simulink model "Modello_attuatore"  (R2023a)
settings: Solver=ode14x  StartTime=0.0  StopTime=3  FixedStep=dt_sim  RelTol=1e-3
values from neighbouring files (symbols this model uses):
  A1_la = 5.710000e-003    (= 0.00571)    [C1_Actuator_1_Data.m]
  A2_la = 5.710000e-003    (= 0.00571)    [C1_Actuator_1_Data.m]
  a_jetpipe_area = 0    [B2_Main_file_Double_Active_Standby_System.m]
  A_svfb = 79.12.*1E-9.*sqrt(pi)    [B2_Main_file_Double_Active_Standby_System.m]
  a_svfb0_1 = 1E-3    (= 0.001)    [B2_Main_file_Double_Active_Standby_System.m]
  a_svfb0_2 = 0    [B2_Main_file_Double_Active_Standby_System.m]
  Afl_sv = dfl_sv^2*pi/4    (= 2.01519637574e-09)    [C1_Actuator_1_Data.m]
  Ag_sv = 18e-6    (= 1.8e-05)    [C1_Actuator_1_Data.m]
  air_gap0_1 = 0    [B2_Main_file_Double_Active_Standby_System.m]
  air_gap_fault_time = 10000    [B2_Main_file_Double_Active_Standby_System.m]
  Asp_sv = 1.35e-5    (= 1.35e-05)    [C1_Actuator_1_Data.m]
  B0_sv = 0.460    (= 0.46)    [C1_Actuator_1_Data.m]
  b_airgap = 0.3    [B2_Main_file_Double_Active_Standby_System.m]
  b_fbspring = 2E-3    (= 0.002)    [B2_Main_file_Double_Active_Standby_System.m]
  b_max = 0*0.0001    (= 0)    [C1_Actuator_1_Data.m]
  beta = 800000000    [D4_Fluid.m]    (also in Rapporto_di_trasmissione.m = acos((L-t.*cos(alpha))./s))
  beta_LVDT = 0    [aggiunte.m]
  bf_sv = 0.45    [C1_Actuator_1_Data.m]
  bsp_sv = 0.25    [C1_Actuator_1_Data.m]
  C_svfb = 1    [B2_Main_file_Double_Active_Standby_System.m]
  Cdmax_sv = 0.7392    [C1_Actuator_1_Data.m]
  Cdmin_sv = 0.6428    [C1_Actuator_1_Data.m]
  CLa = 900000    [aggiunte.m]
  Csa_la = 0.02*sqrt(Ksa_la*Meq_la)    [C1_Actuator_1_Data.m]
  Del_on = 1    [B2_Main_file_Double_Active_Standby_System.m]
  demag0_1 = 0    [B2_Main_file_Double_Active_Standby_System.m]
  dfl_sv = 5.0654e-5    (= 5.0654e-05)    [C1_Actuator_1_Data.m]
  dt_sim = 1e-5    (= 1e-05)    [B2_Main_file_Double_Active_Standby_System.m]
  enable_jetpipe_distorsion = 0    [B2_Main_file_Double_Active_Standby_System.m]
  F_att_sv = 4    [C1_Actuator_1_Data.m]
  FH = FH+0.175*pi*Dd_se(ii)*(-0.884+0.0206*Hs_se(ii)-0.0001*(Hs_se(ii))^2)*Tw_se(ii)    [D2_Data_seal.m]
  first_cycle = 0    [B2_Main_file_Double_Active_Standby_System.m]
  flight_hours = 8    [B2_Main_file_Double_Active_Standby_System.m]
  g_sv = G_sv/l0_sv    (= 0)    [C1_Actuator_1_Data.m]
  Gamma_la = 1.667e4    (= 16670)    [C1_Actuator_1_Data.m]
  gap_ms = 0    [C1_Actuator_1_Data.m]
  Gq_sv = 0.069    [C1_Actuator_1_Data.m]
  Gust_stiffness_jetpipe = 1e8    (= 100000000)    [B2_Main_file_Double_Active_Standby_System.m]
  Gust_threshold = 10000    [B2_Main_file_Double_Active_Standby_System.m]
  h_fbspring = 1E-3    (= 0.001)    [B2_Main_file_Double_Active_Standby_System.m]
  h_sv = H_sv/l0_sv    (= 0)    [C1_Actuator_1_Data.m]
  hr_sv = 6e-6    (= 6e-06)    [C1_Actuator_1_Data.m]
  hyd_fluid_repl = 20    [B2_Main_file_Double_Active_Standby_System.m]
  imax_sv = 8e-3    (= 0.008)    [C1_Actuator_1_Data.m]
  Ja_sv = 1.0575e-5    (= 1.0575e-05)    [C1_Actuator_1_Data.m]
  jetpipe_initialpos = 0    [B2_Main_file_Double_Active_Standby_System.m]
  jetpipe_passage_area = 1    [B2_Main_file_Double_Active_Standby_System.m]
  k_airgap = 0.5/100*0.01    (= 5e-05)    [B2_Main_file_Double_Active_Standby_System.m]
  k_c0_jetpipe_area = 0*1e-1    (= 0)    [B2_Main_file_Double_Active_Standby_System.m]
  k_sv = mup_sv*Vp_sv/(2*B0_sv*l0_sv)-1    (= 16.0383594613)    [C1_Actuator_1_Data.m]
  Kf_sv = 301.6    [C1_Actuator_1_Data.m]
  KFPi = zeros(m,1)    [D2_Data_seal.m]
  Kli1 = 0    [C1_Actuator_1_Data.m]
  Kli2 = 0    [C1_Actuator_1_Data.m]
  Ksa_la = 12480000    [C1_Actuator_1_Data.m]
  Kw_sv = 14.5    [C1_Actuator_1_Data.m]
  l0_sv = 0.5e-3    (= 0.0005)    [C1_Actuator_1_Data.m]
  L_c = imax_sv    (= 0.008)    [C1_Actuator_1_Data.m]
  L_la1 = 0.059900    (= 0.0599)    [C1_Actuator_1_Data.m]
  L_la2 = 0.084800    (= 0.0848)    [C1_Actuator_1_Data.m]
  la_sv = 41e-3    (= 0.041)    [C1_Actuator_1_Data.m]
  lambda_LVDT = 0*0.005*1.5    (= 0)    [aggiunte.m]
  lf = 0.025    [C1_Actuator_1_Data.m]    (also in C2_Actuator_2_Data.m)
  LVDTsize0 = 1    [aggiunte.m]
  m_thermal = 0    [B2_Main_file_Double_Active_Standby_System.m]
  Mcyl_la = 30.425550    (= 30.42555)    [C1_Actuator_1_Data.m]
  Mrod_la = 11.313490    (= 11.31349)    [C1_Actuator_1_Data.m]
  msp_sv = 0.005    [C1_Actuator_1_Data.m]
  mua_sv = 4*pi/1e7    (= 1.25663706144e-06)    [C1_Actuator_1_Data.m]
  mup_sv = 1.1*4*pi/1e7    (= 1.38230076758e-06)    [C1_Actuator_1_Data.m]
  n1_sv = 1140    [C1_Actuator_1_Data.m]
  n2_sv = 1140    [C1_Actuator_1_Data.m]
  n_svfb = 3    [B2_Main_file_Double_Active_Standby_System.m]
  null_shift = -1+2*rand(1,1)    [B2_Main_file_Double_Active_Standby_System.m]
  null_shift_sign = -1+((-1+2*rand(1,1))>=0)*2    [B2_Main_file_Double_Active_Standby_System.m]
  OV_R1 = 0*2.344e-05    (= 0)    [C1_Actuator_1_Data.m]
  OV_R2 = 0*2.344e-05    (= 0)    [C1_Actuator_1_Data.m]
  OV_S1 = 0*2.344e-05    (= 0)    [C1_Actuator_1_Data.m]
  OV_S2 = 0*2.344e-05    (= 0)    [C1_Actuator_1_Data.m]
  P01_la = Pmean-DP_eq    [C1_Actuator_1_Data.m]
  P02_la = Pmean+DP_eq    [C1_Actuator_1_Data.m]
  perc_passage_area0_1 = 0    [B2_Main_file_Double_Active_Standby_System.m]
  Pocl_A = 0    [C1_Actuator_1_Data.m]
  Pocl_B = 0    [C1_Actuator_1_Data.m]
  Pr = 600000    [B2_Main_file_Double_Active_Standby_System.m]
  Ps = 35000000    [B2_Main_file_Double_Active_Standby_System.m]
  R_th1 = 0    [B2_Main_file_Double_Active_Standby_System.m]
  Remax_sv = 5000    [C1_Actuator_1_Data.m]
  Resistance = 1    [C1_Actuator_1_Data.m]
  rj_sv = 1e-6    (= 1e-06)    [C1_Actuator_1_Data.m]
  Rp02_svspring = 1014    [B2_Main_file_Double_Active_Standby_System.m]
  sigma_0LVDT = 0*0.01*1.5*5    (= 0)    [aggiunte.m]
  ST_AD = ceil(10000/fs_AD)/10000    [C1_Actuator_1_Data.m]
  sv_crackON1 = 0    [B2_Main_file_Double_Active_Standby_System.m]
  sv_crackON2 = 0    [B2_Main_file_Double_Active_Standby_System.m]
  T0 = 0    [aggiunte.m]
  tau_w1 = 0    [B2_Main_file_Double_Active_Standby_System.m]
  Temperature_threshold = 0    [B2_Main_file_Double_Active_Standby_System.m]
  V01_la = (Vm_la1+A1_la*(L_la1+x0_la))    (= 0.00040017393)    [C1_Actuator_1_Data.m]
  V02_la = (Vm_la2+A2_la*(L_la2-x0_la))    (= 0.00056652336)    [C1_Actuator_1_Data.m]
  Voltage_com = Resistance    (= 1)    [C1_Actuator_1_Data.m]
  Vp_sv = 5.67e3    (= 5670)    [C1_Actuator_1_Data.m]
  w_fb = 310    [C1_Actuator_1_Data.m]
  w_sv = W_sv/l0_sv    (= 0)    [C1_Actuator_1_Data.m]
  wsp_sv = 0.009334348785340    (= 0.00933434878534)    [C1_Actuator_1_Data.m]
  x0_la = 0    [C1_Actuator_1_Data.m]
  xf_sv_max = 3.05e-5    (= 3.05e-05)    [C1_Actuator_1_Data.m]
  xmax_sb = 5.5e-3    (= 0.0055)    [C1_Actuator_1_Data.m]
  xspmax_sv = 0.001250    (= 0.00125)    [C1_Actuator_1_Data.m]
  z_fb = 0.5    [C1_Actuator_1_Data.m]
undefined symbols (not defined in the file or in its folder): magnitude, Newton, R_sp_C, Raphson
libraries: simulink x13
(part 2 of 3)

== system Modello_attuatore/Actuation System/Servovalve/Spool/orifice2R-resistences ==
  In3 : Inport
  In6 : Inport  Port=2
  In4 : Inport  Port=3
  >=0 : Saturate  UpperLimit=0  LowerLimit=-inf
  >=1 : Saturate  UpperLimit=inf  LowerLimit=0
  Abs : Abs  SaturateOnIntegerOverflow=off
  Abs1 : Abs  SaturateOnIntegerOverflow=off
  Add3 : Sum  Inputs=-|+
  Add4 : Sum  Inputs=+|+
  Cd : Subsystem
  Demux : Demux  Outputs=2
  Fcn : Fcn  Expr=12*u(2)*u(1)/(2.5*wsp_sv*hr_sv^3)
  Fcn1 : Fcn  Expr=u(1)/(2*u(2)^2*u(3)^2)
  Math Function2 : Math  Operator=magnitude^2  SignedPower=on
  Math Function3 : Math  Operator=magnitude^2  SignedPower=on
  Mux : Mux  Inputs=2
  Mux1 : Mux  Inputs=3
  Product : Product  RndMeth=Zero
  Sqrt1 : Sqrt  AlgorithmType=Newton-Raphson
  gioco radiale : Constant  Value=hr_sv
  gioco radiale1 : Constant  Value=wsp_sv
  ricoprimento : Constant  Value=OV_R2
  Out1 : Outport
  Out2 : Outport  Port=2
  wires:
  Mux/1 -> Fcn/1
  Mux1/1 -> Fcn1/1
  Fcn1/1 -> Out1/1  "R_AR2"
  Demux/2 -> Mux/2  "mu [Pa s]"
  Cd/1(Out3) -> Mux1/2  "Cd"
  In4/1 -> Abs/1  "Q2R[m3/s]"
  Demux/1 -> Mux1/1  "ro [kg/m3]"
  In6/1 -> Demux/1  "ro;mu"
  ricoprimento/1 -> Add3/1
  In3/1 -> Add3/2  "xs[m]"
  Abs/1 -> Cd/1(In2)
  gioco radiale/1 -> Math Function2/1  "hr[m]"
  Add3/1 -> >=1/1, >=0/1  "x[m]"
  >=0/1 -> Abs1/1
  Add4/1 -> Sqrt1/1
  Math Function3/1 -> Add4/1
  Math Function2/1 -> Add4/2
  gioco radiale1/1 -> Product/2  "w[m]"
  Abs1/1 -> Mux/1
  >=1/1 -> Math Function3/1, Cd/2(In1)
  Sqrt1/1 -> Product/1, Cd/3(In3)  "l[m]"
  Product/1 -> Mux1/3  "A [m2]"
  Fcn/1 -> Out2/1  "R_CR2"

== system Modello_attuatore/Actuation System/Servovalve/Spool/orifice2S-resistences ==
  In3 : Inport
  In6 : Inport  Port=2
  In4 : Inport  Port=3
  >=0 : Saturate  UpperLimit=inf  LowerLimit=0
  >=1 : Saturate  UpperLimit=0  LowerLimit=-inf
  Abs : Abs  SaturateOnIntegerOverflow=off
  Abs1 : Abs  SaturateOnIntegerOverflow=off
  Add3 : Sum  Inputs=+|+
  Add4 : Sum  Inputs=+|+
  Cd : Subsystem
  Demux : Demux  Outputs=2
  Fcn : Fcn  Expr=12*u(2)*u(1)/(2.5*wsp_sv*hr_sv^3)
  Fcn1 : Fcn  Expr=u(1)/(2*u(2)^2*u(3)^2)
  Math Function2 : Math  Operator=magnitude^2  SignedPower=on
  Math Function3 : Math  Operator=magnitude^2  SignedPower=on
  Mux : Mux  Inputs=2
  Mux1 : Mux  Inputs=3
  Product : Product  RndMeth=Zero
  Sqrt1 : Sqrt  AlgorithmType=Newton-Raphson
  gioco radiale : Constant  Value=hr_sv
  gioco radiale1 : Constant  Value=wsp_sv
  ricoprimento : Constant  Value=OV_S2
  Out1 : Outport
  Out2 : Outport  Port=2
  wires:
  Mux/1 -> Fcn/1
  Mux1/1 -> Fcn1/1
  Fcn1/1 -> Out1/1  "R_AS2"
  Demux/2 -> Mux/2  "mu [Pa s]"
  Cd/1(Out3) -> Mux1/2  "Cd"
  In4/1 -> Abs/1  "Q2S[m3/s]"
  Demux/1 -> Mux1/1  "ro [kg/m3]"
  In6/1 -> Demux/1  "ro;mu"
  ricoprimento/1 -> Add3/1
  In3/1 -> Add3/2  "xs[m]"
  Abs/1 -> Cd/1(In2)
  gioco radiale/1 -> Math Function2/1  "hr[m]"
  Add3/1 -> >=1/1, >=0/1  "x[m]"
  >=0/1 -> Abs1/1
  Add4/1 -> Sqrt1/1
  Math Function3/1 -> Add4/1
  Math Function2/1 -> Add4/2
  gioco radiale1/1 -> Product/2  "w[m]"
  Abs1/1 -> Mux/1
  >=1/1 -> Math Function3/1, Cd/2(In1)
  Sqrt1/1 -> Product/1, Cd/3(In3)  "l[m]"
  Product/1 -> Mux1/3  "A [m2]"
  Fcn/1 -> Out2/1  "R_CS2"

== system Modello_attuatore/Actuation System/Servovalve/Spool/orificeS1-flow ==
  In4 : Inport
  In2 : Inport  Port=2
  In1 : Inport  Port=3
  Gain : Gain  Gain=4  SaturateOnIntegerOverflow=on  OutDataTypeStr=Inherit: Same as input  ParamDataTypeStr=Inherit: Same as input
  Gain1 : Gain  Gain=2  SaturateOnIntegerOverflow=on  OutDataTypeStr=Inherit: Same as input  ParamDataTypeStr=Inherit: Same as input
  Math Function : Math  Operator=sqrt  SignedPower=on
  Math Function1 : Math  Operator=magnitude^2  SignedPower=on
  Product : Product  Inputs=3  SaturateOnIntegerOverflow=on  OutDataTypeStr=Inherit: Same as first input
  Product1 : Product  Inputs=*/  SaturateOnIntegerOverflow=on  OutDataTypeStr=Inherit: Same as first input
  Product2 : Product  SaturateOnIntegerOverflow=on  OutDataTypeStr=Inherit: Same as first input
  Sign : Signum
  Sum : Sum  Inputs=|++  SaturateOnIntegerOverflow=on
  Sum1 : Sum  Inputs=|+-  SaturateOnIntegerOverflow=on
  Out1 : Outport
  wires:
  Sign/1 -> Product/1, Product2/1
  In4/1 -> Product/2, Sign/1  "dP[Pa]"
  In2/1 -> Gain1/1, Product/3  "R_AS1"
  Product/1 -> Gain/1
  Gain/1 -> Sum/1
  Math Function1/1 -> Sum/2
  Sum/1 -> Math Function/1
  Math Function/1 -> Sum1/1
  Sum1/1 -> Product1/1
  Gain1/1 -> Product1/2
  Product1/1 -> Product2/2
  In1/1 -> Sum1/2, Math Function1/1  "R_CS1"
  Product2/1 -> Out1/1  "Q_1S[m3/s]"

== system Modello_attuatore/Actuation System/Servovalve/Spool/orificeS2-flow ==
  In4 : Inport
  In1 : Inport  Port=2
  In2 : Inport  Port=3
  Gain : Gain  Gain=4  SaturateOnIntegerOverflow=on  OutDataTypeStr=Inherit: Same as input  ParamDataTypeStr=Inherit: Same as input
  Gain1 : Gain  Gain=2  SaturateOnIntegerOverflow=on  OutDataTypeStr=Inherit: Same as input  ParamDataTypeStr=Inherit: Same as input
  Math Function : Math  Operator=sqrt  SignedPower=on
  Math Function1 : Math  Operator=magnitude^2  SignedPower=on
  Product : Product  Inputs=3  SaturateOnIntegerOverflow=on  OutDataTypeStr=Inherit: Same as first input
  Product1 : Product  Inputs=*/  SaturateOnIntegerOverflow=on  OutDataTypeStr=Inherit: Same as first input
  Product2 : Product  SaturateOnIntegerOverflow=on  OutDataTypeStr=Inherit: Same as first input
  Sign : Signum
  Sum : Sum  Inputs=|++  SaturateOnIntegerOverflow=on
  Sum1 : Sum  Inputs=|+-  SaturateOnIntegerOverflow=on
  Out4 : Outport
  wires:
  Product2/1 -> Out4/1  "Q_2S[m3/s]"
  In2/1 -> Math Function1/1, Sum1/2  "R_CR2"
  Product1/1 -> Product2/2
  Gain1/1 -> Product1/2
  Sum1/1 -> Product1/1
  Math Function/1 -> Sum1/1
  Sum/1 -> Math Function/1
  Math Function1/1 -> Sum/2
  Gain/1 -> Sum/1
  Product/1 -> Gain/1
  In1/1 -> Product/3, Gain1/1  "R_AS2"
  In4/1 -> Product/2, Sign/1  "dP[Pa]"
  Sign/1 -> Product2/1, Product/1

== system Modello_attuatore/Actuation System/Actuator/Rod/Double Integrator/Limit ==
  In2 : Inport
  In1 : Inport  Port=2
  Constant : Constant
  Constant1 : Constant  Value=-1
  Constant2 : Constant  Value=0
  Constant3 : Constant  Value=0
  Logical Operator : Logic  AllPortsSameDT=off
  Logical Operator1 : Logic  AllPortsSameDT=off
  Logical Operator2 : Logic  Operator=NOR  AllPortsSameDT=off
  Product : Product  RndMeth=Zero
  Relational Operator : RelationalOperator  Operator=>  OutDataTypeStr=boolean  InputSameDT=off
  Relational Operator1 : RelationalOperator  Operator===  OutDataTypeStr=boolean  InputSameDT=off
  Relational Operator2 : RelationalOperator  Operator=<  OutDataTypeStr=boolean  InputSameDT=off
  Relational Operator3 : RelationalOperator  Operator===  OutDataTypeStr=boolean  InputSameDT=off
  Out2 : Outport
  wires:
  In2/1 -> Relational Operator/1, Product/1, Relational Operator2/1  "xrod_dd [m/s2]"
  In1/1 -> Relational Operator3/1, Relational Operator1/1  "limit xrod"
  Constant3/1 -> Relational Operator/2
  Constant/1 -> Relational Operator1/2
  Constant1/1 -> Relational Operator3/2
  Constant2/1 -> Relational Operator2/2
  Relational Operator/1 -> Logical Operator/1
  Relational Operator1/1 -> Logical Operator/2
  Relational Operator3/1 -> Logical Operator1/1
  Relational Operator2/1 -> Logical Operator1/2
  Logical Operator/1 -> Logical Operator2/1
  Logical Operator1/1 -> Logical Operator2/2
  Logical Operator2/1 -> Product/2
  Product/1 -> Out2/1  "xrod_dd [m2/s]"

== system Modello_attuatore/Actuation System/Actuator/Rod/Friction1/FP ==
  In3 : Inport
  Abs : Abs  SaturateOnIntegerOverflow=off
  Abs1 : Abs  SaturateOnIntegerOverflow=off
  Abs2 : Abs  SaturateOnIntegerOverflow=off
  Add1 : Sum  Inputs=+|+
  Constant1 : Constant  Value=KFPi
  Constant2 : Constant  Value=FH
  Demux : Demux  Outputs=2
  Display : Display
  Display1 : Display
  Mux6 : Mux  Inputs=2
  P1-Patm : Fcn  Expr=(u(1)*1e-6)^0.61
  P2-Patm : Fcn  Expr=(u(1)*1e-6)^0.61
  Product3 : Product  RndMeth=Zero
  Scope3 : Scope
  Scope4 : Scope
  Sum of Elements : Sum  Inputs=+
  Vector Concatenate1 : Concatenate  NumInputs=3  ConcatenateDimension=2
  abs(P1-P2) : Fcn  Expr=(abs(u(1)-u(2))*1e-6)^0.61
  Out4 : Outport
  wires:
  Constant2/1 -> Display1/1, Add1/2
  Add1/1 -> Out4/1, Scope3/1  "FP+FH"
  Sum of Elements/1 -> Add1/1, Display/1  "FP"
  Abs/1 -> abs(P1-P2)/1
  Product3/1 -> Sum of Elements/1  "KFPi"
  Constant1/1 -> Product3/2
  Vector Concatenate1/1 -> Scope4/1, Product3/1
  abs(P1-P2)/1 -> Vector Concatenate1/3
  P2-Patm/1 -> Vector Concatenate1/2
  Demux/2 -> Mux6/2, Abs2/1  "P2"
  Demux/1 -> Mux6/1, Abs1/1  "P1"
  P1-Patm/1 -> Vector Concatenate1/1
  Mux6/1 -> Abs/1
  In3/1 -> Demux/1  "P"
  Abs1/1 -> P1-Patm/1
  Abs2/1 -> P2-Patm/1

== system Modello_attuatore/Actuation System/Actuator/Sleeve/Backlash/No Backlash ==
  In1 : Inport
  In2 : Inport  Port=2
  Action Port : ActionPort  PropagateVarSize=During execution  ActionPortLabel=if(u1<=1e-10)
  Add4 : Sum  Inputs=+|+
  Cs_shaft [Nm/(rad/s)] : Gain  Gain=Csa_la
  Ks_shaft [Nm/rad] : Gain  Gain=Ksa_la
  Out3 : Outport
  wires:
  Ks_shaft [Nm/rad]/1 -> Add4/1
  Cs_shaft [Nm/(rad/s)]/1 -> Add4/2
  Add4/1 -> Out3/1
  In1/1 -> Ks_shaft [Nm/rad]/1
  In2/1 -> Cs_shaft [Nm/(rad/s)]/1

== system Modello_attuatore/Actuation System/Actuator/Sleeve/Backlash/No contact ==
  In2 : Inport
  In3 : Inport  Port=2
  Action Port : ActionPort  PropagateVarSize=During execution  ActionPortLabel=else
  Add4 : Sum  Inputs=+|+
  no torque : Gain  Gain=0
  Out3 : Outport
  wires:
  no torque/1 -> Out3/1
  In2/1 -> Add4/1
  In3/1 -> Add4/2
  Add4/1 -> no torque/1

== system Modello_attuatore/Actuation System/Actuator/Sleeve/Backlash/phi diff > max backlash ==
  In2 : Inport
  In3 : Inport  Port=2
  Action Port : ActionPort  PropagateVarSize=During execution  ActionPortLabel=elseif(u2>u3)
  Add1 : Sum  Inputs=+|-
  Add2 : Sum  Inputs=+|+
  Add4 : Sum  Inputs=+|+
  Compare To Zero : simulink/Logic and Bit Operations/Compare To Zero  relop=<=  OutDataTypeStr=uint8
  Constant : Constant  Value=0
  Constant2 : Constant  Value=b_max/2
  Cs_shaft [Nm/(rad/s)] : Gain  Gain=Csa_la
  Ks_shaft [Nm/rad] : Gain  Gain=Ksa_la
  MinMax : MinMax  Inputs=2
  Switch : Switch  Criteria=u2 > Threshold  SaturateOnIntegerOverflow=off  InputSameDT=off
  Out1 : Outport
  wires:
  Ks_shaft [Nm/rad]/1 -> Add4/1, MinMax/1, Add2/1
  Cs_shaft [Nm/(rad/s)]/1 -> Add4/2, MinMax/2
  In3/1 -> Cs_shaft [Nm/(rad/s)]/1
  In2/1 -> Add1/1
  Constant2/1 -> Add1/2
  Add1/1 -> Ks_shaft [Nm/rad]/1
  Compare To Zero/1 -> Switch/2
  Constant/1 -> Switch/1
  Add4/1 -> Compare To Zero/1
  MinMax/1 -> Add2/2
  Add2/1 -> Switch/3
  Switch/1 -> Out1/1  "Force [N]"

== system Modello_attuatore/Actuation System/Actuator/Sleeve/Backlash/phi diff< min backlash ==
  In2 : Inport
  In3 : Inport  Port=2
  Action Port : ActionPort  PropagateVarSize=During execution  ActionPortLabel=elseif( u2<u4)
  Add1 : Sum  Inputs=+|-
  Add2 : Sum  Inputs=+|+
  Add4 : Sum  Inputs=+|+
  Compare To Zero : simulink/Logic and Bit Operations/Compare To Zero  relop=>=  OutDataTypeStr=uint8
  Constant : Constant  Value=0
  Constant1 : Constant  Value=-b_max/2
  Cs_shaft [Nm/(rad/s)] : Gain  Gain=Csa_la
  Ks_shaft [Nm/rad] : Gain  Gain=Ksa_la
  MinMax : MinMax  Function=max  Inputs=2
  Switch : Switch  Criteria=u2 > Threshold  SaturateOnIntegerOverflow=off  InputSameDT=off
  Out1 : Outport
  wires:
  Ks_shaft [Nm/rad]/1 -> Add4/1, MinMax/1, Add2/1
  Cs_shaft [Nm/(rad/s)]/1 -> Add4/2, MinMax/2
  In3/1 -> Cs_shaft [Nm/(rad/s)]/1
  In2/1 -> Add1/1
  Constant1/1 -> Add1/2
  Add1/1 -> Ks_shaft [Nm/rad]/1
  Compare To Zero/1 -> Switch/2
  Constant/1 -> Switch/1
  Add4/1 -> Compare To Zero/1
  MinMax/1 -> Add2/2
  Add2/1 -> Switch/3
  Switch/1 -> Out1/1  "Force [N]"

== system Modello_attuatore/Actuation System/Servovalve/Servovalve Dynamic/Crack propagation/Bending (normal) stress computation ==
  Tb [Nm] : Inport
  Crack_size[mm] : Inport  Port=2
  Add : Sum  Inputs=-+
  Constant : Constant  Value=b_fbspring*1000
  Constant1 : Constant  Value=h_fbspring*1000
  Divide : Product  Inputs=*/*
  Divide1 : Product  Inputs=**
  Fcn : Fcn  Expr=(u(1)^3)
  Gain : Gain  Gain=0.5
  Gain1 : Gain
  Gain2 : Gain  Gain=1/12
  Gain3 : Gain  Gain=1000
  Saturation : Saturate  UpperLimit=Inf  LowerLimit=1E-5
  sigma [MPa] : Outport
  wires:
  Tb [Nm]/1 -> Gain3/1
  Add/1 -> Fcn/1, Gain/1
  Divide/1 -> Gain1/1
  Crack_size[mm]/1 -> Add/1
  Constant1/1 -> Add/2
  Gain/1 -> Divide/3
  Gain1/1 -> sigma [MPa]/1
  Fcn/1 -> Gain2/1  "Wbend"
  Gain2/1 -> Divide1/2
  Constant/1 -> Divide1/1
  Divide1/1 -> Saturation/1
  Saturation/1 -> Divide/2
  Gain3/1 -> Divide/1

== system Modello_attuatore/Actuation System/Servovalve/Servovalve Dynamic/Crack propagation/Enabled Subsystem ==
  max,min : Inport
  Enable : EnablePort  StatesWhenEnabling=reset  ShowOutputPort=on
  Abs : Abs  SaturateOnIntegerOverflow=off
  Add : Sum  Inputs=+-
  Add1 : Sum  Inputs=+-
  Demux : Demux  Outputs=2
  Saturation : Saturate  UpperLimit=inf  LowerLimit=0
  Saturation1 : Saturate  UpperLimit=0  LowerLimit=-inf
  Saturation2 : Saturate  UpperLimit=inf  LowerLimit=0
  Saturation3 : Saturate  UpperLimit=0  LowerLimit=-inf
  DeltaS_side1 : Outport
  DeltaS_side2 : Outport  Port=2
  Reset_minmax : Outport  Port=3
  wires:
  max,min/1 -> Demux/1
  Demux/2 -> Saturation/1, Saturation3/1
  Demux/1 -> Saturation1/1, Saturation2/1
  Saturation/1 -> Add/2
  Saturation2/1 -> Add/1
  Saturation3/1 -> Add1/2
  Add/1 -> DeltaS_side1/1
  Add1/1 -> Abs/1
  Enable/1 -> Reset_minmax/1
  Abs/1 -> DeltaS_side2/1
  Saturation1/1 -> Add1/1

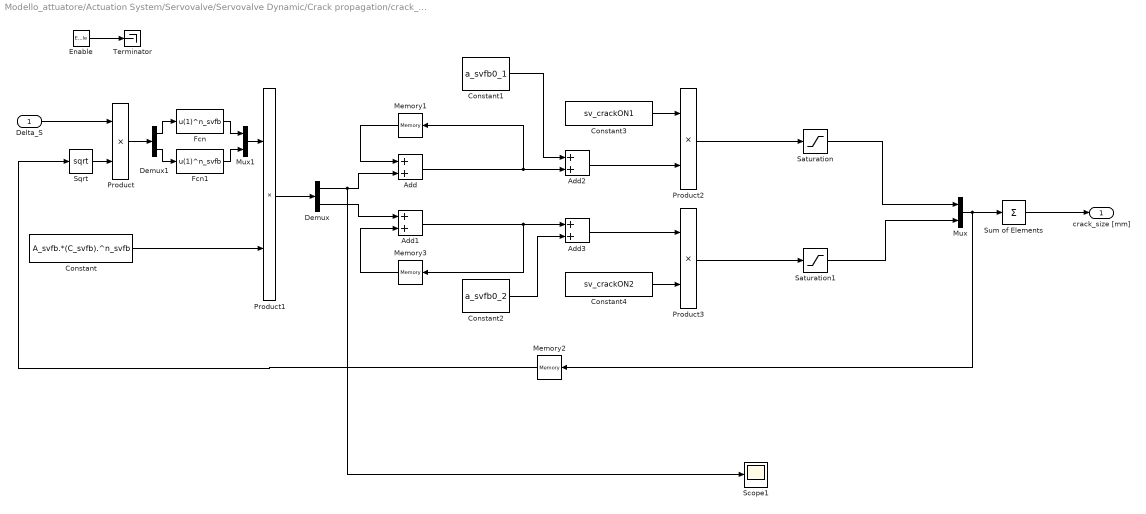
== system Modello_attuatore/Actuation System/Servovalve/Servovalve Dynamic/Crack propagation/crack_size calculation ==
  Delta_S : Inport
  Enable : EnablePort  ShowOutputPort=on
  Add{,1..3} (4 alike) : Sum
  Constant : Constant  Value=A_svfb.*(C_svfb).^n_svfb
  Constant1 : Constant  Value=a_svfb0_1
  Constant2 : Constant  Value=a_svfb0_2
  Constant3 : Constant  Value=sv_crackON1
  Constant4 : Constant  Value=sv_crackON2
  Demux : Demux  Outputs=2
  Demux1 : Demux  Outputs=2
  Fcn : Fcn  Expr=u(1)^n_svfb
  Fcn1 : Fcn  Expr=u(1)^n_svfb
  Memory1 : Memory
  Memory2 : Memory  InitialCondition=[a_svfb0_1; a_svfb0_2]
  Memory3 : Memory
  Mux : Mux  Inputs=2
  Mux1 : Mux  Inputs=2
  Product{,1..3} (4 alike) : Product
  Saturation : Saturate  UpperLimit=h_fbspring*1000  LowerLimit=0
  Saturation1 : Saturate  UpperLimit=h_fbspring*1000  LowerLimit=0
  Scope1 : Scope
  Sqrt : Sqrt
  Sum of Elements : Sum  Inputs=+
  Terminator : Terminator
  crack_size [mm] : Outport
  wires:
  Delta_S/1 -> Product/1
  Sqrt/1 -> Product/2
  Constant/1 -> Product1/2
  Product1/1 -> Demux/1
  Demux/2 -> Add1/1
  Add/1 -> Memory1/1, Add2/2
  Add1/1 -> Memory3/1, Add3/1
  Constant1/1 -> Add2/1
  Constant2/1 -> Add3/2
  Add2/1 -> Product2/2
  Constant3/1 -> Product2/1
  Constant4/1 -> Product3/2
  Add3/1 -> Product3/1
  Product2/1 -> Saturation/1
  Product3/1 -> Saturation1/1
  Product/1 -> Demux1/1
  Demux1/1 -> Fcn/1
  Demux1/2 -> Fcn1/1
  Fcn/1 -> Mux1/1
  Fcn1/1 -> Mux1/2
  Sum of Elements/1 -> crack_size [mm]/1
  Memory1/1 -> Add/1
  Memory3/1 -> Add1/2
  Mux1/1 -> Product1/1
  Mux/1 -> Memory2/1, Sum of Elements/1
  Memory2/1 -> Sqrt/1
  Saturation/1 -> Mux/1
  Saturation1/1 -> Mux/2
  Enable/1 -> Terminator/1
  Demux/1 -> Scope1/1, Add/2

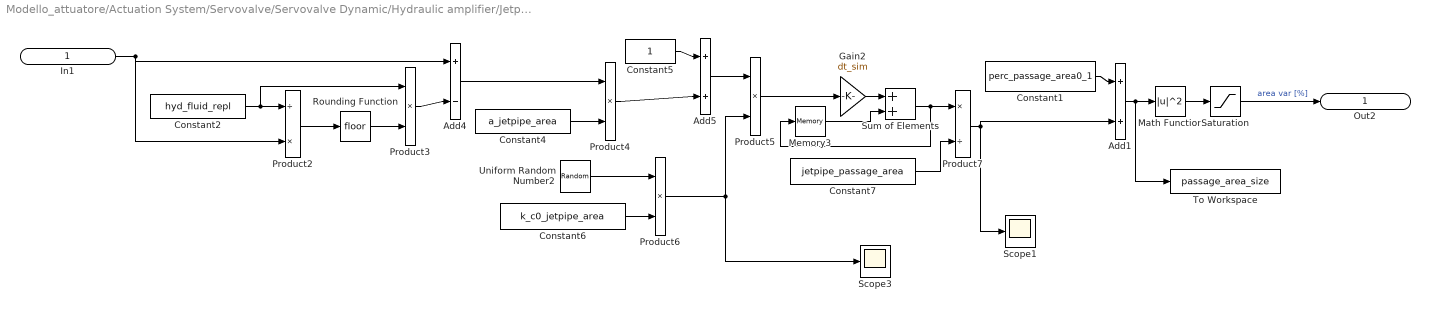
== system Modello_attuatore/Actuation System/Servovalve/Servovalve Dynamic/Hydraulic amplifier/Jetpipe area occlusion ==
  In1 : Inport
  Add1 : Sum  Inputs=+|+
  Add4 : Sum  Inputs=+|-
  Add5 : Sum  Inputs=+|+
  Constant1 : Constant  Value=perc_passage_area0_1
  Constant2 : Constant  Value=hyd_fluid_repl
  Constant4 : Constant  Value=a_jetpipe_area
  Constant5 : Constant
  Constant6 : Constant  Value=k_c0_jetpipe_area
  Constant7 : Constant  Value=jetpipe_passage_area
  Gain2 : Gain  Gain=dt_sim
  Math Function : Math  Operator=magnitude^2  SignedPower=on
  Memory3 : Memory
  Product2 : Product  Inputs=/*  SaturateOnIntegerOverflow=on  OutDataTypeStr=Inherit: Same as first input
  Product{3..6} (4 alike) : Product  SaturateOnIntegerOverflow=on  OutDataTypeStr=Inherit: Same as first input
  Product7 : Product  Inputs=*/  SaturateOnIntegerOverflow=on  OutDataTypeStr=Inherit: Same as first input
  Rounding Function : Rounding
  Saturation : Saturate  UpperLimit=0.8  LowerLimit=0
  Scope1 : Scope
  Scope3 : Scope
  Sum of Elements : Sum
  To Workspace : ToWorkspace  VariableName=passage_area_size  SaveFormat=Structure With Time  SampleTime=-1
  Uniform Random Number2 : UniformRandomNumber  Minimum=1  Maximum=5
  Out2 : Outport
  wires:
  In1/1 -> Product2/2, Add4/1
  Product2/1 -> Rounding Function/1
  Constant2/1 -> Product2/1, Product3/1
  Rounding Function/1 -> Product3/2
  Product3/1 -> Add4/2
  Add4/1 -> Product4/1
  Product4/1 -> Add5/2
  Constant5/1 -> Add5/1
  Constant4/1 -> Product4/2
  Add5/1 -> Product5/1
  Constant6/1 -> Product6/2
  Uniform Random Number2/1 -> Product6/1
  Product6/1 -> Product5/2, Scope3/1
  Gain2/1 -> Sum of Elements/1
  Product5/1 -> Gain2/1
  Sum of Elements/1 -> Memory3/1, Product7/1
  Memory3/1 -> Sum of Elements/2
  Constant7/1 -> Product7/2
  Product7/1 -> Scope1/1, Add1/2
  Saturation/1 -> Out2/1  "area var [%]"
  Add1/1 -> Math Function/1, To Workspace/1
  Constant1/1 -> Add1/1
  Math Function/1 -> Saturation/1

== system Modello_attuatore/Actuation System/Servovalve/Servovalve Dynamic/Hydraulic amplifier/Ugello A ==
  In4 : Inport
  In2 : Inport  Port=2
  In1 : Inport  Port=3
  In3 : Inport  Port=4
  In5 : Inport  Port=5
  Add1 : Sum  Inputs=+|-
  Add2 : Sum  Inputs=+|+
  Constant : Fcn  Expr=((u(2)-(u(4)*u(2)))-(u(3)+Pocl_A))/2+(u(3)+Pocl_A)
  Gain1 : Gain  Gain=Asp_sv/Gq_sv
  Mux2 : Mux
  Saturation2 : Saturate  UpperLimit=Ps  LowerLimit=Pr
  tt : Fcn  Expr=u(1)*((u(2)-(u(4)*u(2)))-(u(3)+Pocl_A))/(2*xf_sv_max)
  PA : Outport
  wires:
  Add2/1 -> Saturation2/1
  Saturation2/1 -> PA/1  "PA"
  In2/1 -> Gain1/1  "dxs[m/s]"
  In4/1 -> Add1/1  "xf[m]"
  Gain1/1 -> Add1/2
  Add1/1 -> Mux2/1
  Mux2/1 -> tt/1, Constant/1
  tt/1 -> Add2/1
  Constant/1 -> Add2/2
  In1/1 -> Mux2/2
  In3/1 -> Mux2/3
  In5/1 -> Mux2/4

== system Modello_attuatore/Actuation System/Servovalve/Servovalve Dynamic/Hydraulic amplifier/Ugello B ==
  In5 : Inport
  In3 : Inport  Port=2
  In1 : Inport  Port=3
  In2 : Inport  Port=4
  In4 : Inport  Port=5
  Add1 : Sum  Inputs=+|-
  Add2 : Sum  Inputs=+|+
  Constant : Fcn  Expr=((u(2)-(u(4)*u(2)))-(u(3)+Pocl_B))/2+(u(3)+Pocl_B)
  Gain1 : Gain  Gain=Asp_sv/Gq_sv
  Mux1 : Mux
  Saturation2 : Saturate  UpperLimit=Ps  LowerLimit=Pr
  tt : Fcn  Expr=u(1)*(-((u(2)-(u(4)*u(2)))-(u(3)+Pocl_B))/(2*xf_sv_max))
  PB : Outport
  wires:
  In2/1 -> Gain1/1  "dxs[m/s]"
  In4/1 -> Add1/1  "xf[m]"
  Gain1/1 -> Add1/2
  Saturation2/1 -> PB/1  "PB"
  Add2/1 -> Saturation2/1
  In1/1 -> Mux1/2
  In3/1 -> Mux1/3
  Mux1/1 -> tt/1, Constant/1
  Constant/1 -> Add2/2
  tt/1 -> Add2/1
  Add1/1 -> Mux1/1
  In5/1 -> Mux1/4

== system Modello_attuatore/Actuation System/Servovalve/Servovalve Dynamic/Jet pipe dynamic/Double Integrator ==
  In1 : Inport
  Integrator : Integrator  ExternalReset=either
  Integrator1 : Integrator  LimitOutput=on  UpperSaturationLimit=3.05e-5  LowerSaturationLimit=-3.05e-5  ShowSaturationPort=on
  Limit : Subsystem
  Out1 : Outport
  Out2 : Outport  Port=2
  wires:
  Integrator/1 -> Integrator1/1, Out2/1  "xR_d[m/s]"
  Integrator1/1 -> Out1/1  "xR[m]"
  Limit/1(Out2) -> Integrator/1
  Integrator1/2 -> Integrator/2, Limit/2(In1)  "limit xatt"
  In1/1 -> Limit/1(In2)  "xR_dd[m/s2]"

== system Modello_attuatore/Actuation System/Servovalve/Servovalve Dynamic/Jet pipe dynamic/Jetpipe distorted ==
  In3 : Inport
  In1 : Inport  Port=2
  Add1 : Sum  Inputs=+|+
  Add3 : Sum  Inputs=+|-
  Add4 : Sum  Inputs=+|+
  Compare To Constant : simulink/Logic and Bit Operations/Compare To Constant  relop=>  const=0  OutDataTypeStr=uint8
  Constant1 : Constant  Value=jetpipe_initialpos
  Constant3 : Constant  Value=Gust_threshold
  Gain1 : Gain  Gain=dt_sim
  Gain2 : Gain  Gain=1/Gust_stiffness_jetpipe
  Gain3 : Gain  Gain=enable_jetpipe_distorsion
  Memory3 : Memory
  Product1 : Product  SaturateOnIntegerOverflow=on  OutDataTypeStr=Inherit: Same as first input
  Saturation : Saturate  UpperLimit=0.05*xf_sv_max  LowerLimit=-0.05*xf_sv_max
  Scope1 : Scope
  Scope2 : Scope
  Scope3 : Scope
  Sum of Elements : Sum
  To Workspace : ToWorkspace  VariableName=jetpipe_size  SaveFormat=Structure With Time  SampleTime=-1
  Out2 : Outport
  wires:
  Compare To Constant/1 -> Product1/2, Scope3/1
  Constant3/1 -> Add3/2
  Add3/1 -> Compare To Constant/1, Product1/1
  Product1/1 -> Gain2/1
  In3/1 -> Add3/1
  Sum of Elements/1 -> Memory3/1, Add4/1, Scope2/1
  Memory3/1 -> Sum of Elements/2
  Gain2/1 -> Scope1/1, Gain1/1
  Gain1/1 -> Sum of Elements/1
  Constant1/1 -> Add4/2
  Saturation/1 -> Gain3/1
  Add4/1 -> Saturation/1  "xf[m]"
  In1/1 -> Add1/2
  Add1/1 -> Out2/1
  Gain3/1 -> Add1/1, To Workspace/1

== system Modello_attuatore/Actuation System/Servovalve/Servovalve Dynamic/Spool  dynamic/Double Integrator ==
  In1 : Inport
  In2 : Inport  Port=2
  Abs : Abs  SaturateOnIntegerOverflow=off
  Compare To Constant : simulink/Logic and Bit Operations/Compare To Constant  relop===  const=1  OutDataTypeStr=boolean
  Compare To Constant1 : simulink/Logic and Bit Operations/Compare To Constant  relop===  const=1  OutDataTypeStr=boolean
  Integrator : Integrator  ExternalReset=rising  ShowStatePort=on
  Integrator1 : Integrator  LimitOutput=on  UpperSaturationLimit=xspmax_sv  LowerSaturationLimit=-xspmax_sv  ShowSaturationPort=on
  Limit : Subsystem
  Logical Operator : Logic  Operator=OR  AllPortsSameDT=off  OutDataTypeStr=boolean
  Out1 : Outport
  Out2 : Outport  Port=2
  Out3 : Outport  Port=3
  wires:
  Integrator/1 -> Integrator1/1, Out2/1  "xR_d[m/s]"
  Integrator1/1 -> Out1/1  "xR[m]"
  Limit/1(Out2) -> Integrator/1
  Integrator1/2 -> Limit/2(In1), Abs/1  "limit xatt"
  In1/1 -> Limit/1(In2)  "xR_dd[m/s2]"
  Abs/1 -> Compare To Constant/1
  In2/1 -> Compare To Constant1/1
  Compare To Constant1/1 -> Logical Operator/1
  Compare To Constant/1 -> Logical Operator/2
  Logical Operator/1 -> Integrator/2
  Integrator/State -> Out3/1  "zero-crossing"

== system Modello_attuatore/Actuation System/Servovalve/Servovalve Dynamic/Spool  dynamic/Flow Force ==
  In1 : Inport
  Abs : Abs  SaturateOnIntegerOverflow=off
  Abs1 : Abs  SaturateOnIntegerOverflow=off
  Add : Sum
  Demux : Demux  Outputs=2
  Gain : Gain  Gain=-1
  Mux1 : Mux  Inputs=3
  Product{1..3,5..6} (5 alike) : Product
  Q_max evaluation and flow angle variation : Subsystem
  Scope : Scope
  Scope1 : Scope
  Sign : Signum
  Terminator2 : Terminator
  sqrt(dP*ro) : Fcn  Expr=sqrt(u(3)*(u(1)-u(2)))
  Ffl1+Ffl2 : Outport
  wires:
  [Supply_pressure_var] -> Mux1/1
  [Flow_second_chamber] -> Abs1/1
  [Flow_first_chamber] -> Abs/1
  [Return_pressure_var] -> Mux1/2
  Demux/1 -> Mux1/3
  Product1/1 -> Product5/1
  Abs1/1 -> Q_max evaluation and flow angle variation/3(In3), Product2/2  "Q2 [m3/s]"
  Mux1/1 -> sqrt(dP*ro)/1, Q_max evaluation and flow angle variation/2(In2), Scope1/1  "Ps; Pr; ro"
  Abs/1 -> Product1/1, Q_max evaluation and flow angle variation/1(In1)  "Q1 [m3/s]"
  Product5/1 -> Add/1
  Product6/1 -> Add/2
  Q_max evaluation and flow angle variation/1(cos(teta) of Q1) -> Product1/2
  Q_max evaluation and flow angle variation/2(cos(teta) of Q2) -> Product2/1
  Product2/1 -> Product6/1
  sqrt(dP*ro)/1 -> Product5/2, Product6/2
  In1/1 -> Sign/1
  Product3/1 -> Ffl1+Ffl2/1, Scope/1
  Add/1 -> Product3/2
  Sign/1 -> Gain/1
  Gain/1 -> Product3/1
  Demux/2 -> Terminator2/1
  [Fluid_properties_var] -> Demux/1

== system Modello_attuatore/Actuation System/Servovalve/Servovalve Dynamic/Spool  dynamic/Friction ==
  In1 : Inport
  In2 : Inport  Port=2
  In3 : Inport  Port=3
  Abs : Abs  SaturateOnIntegerOverflow=off
  Add2 : Sum  Inputs=+|-
  Fcoul + viscous friction [N] : Fcn  Expr=((u(2))*(1+(0.5)*exp(-10*abs(u(1)))))+bsp_sv*abs(u(1))
  Hit Crossing : HitCross
  MinMax : MinMax  Inputs=2
  Mux1 : Mux  Inputs=2
  Product : Product  RndMeth=Zero
  Sign1 : Signum
  Sign2 : Signum
  Switch : Switch  Criteria=u2 > Threshold  Threshold=0.0  SaturateOnIntegerOverflow=off  InputSameDT=off
  Switch1 : Switch  Criteria=u2 > Threshold  Threshold=0.0  SaturateOnIntegerOverflow=off  InputSameDT=off
  static friction [N] : Constant  Value=F_att_sv
  Out1 : Outport
  Out2 : Outport  Port=2
  wires:
  Product/1 -> Add2/2  "drag force [N]"
  Switch/1 -> Product/1
  Sign1/1 -> Switch/1
  In1/1 -> Abs/1, Sign1/1, Add2/1
  Add2/1 -> Out1/1  "F_act [N]"
  In2/1 -> Mux1/1, Sign2/1
  Mux1/1 -> Fcoul + viscous friction [N]/1
  Fcoul + viscous friction [N]/1 -> MinMax/2, Switch1/3
  Hit Crossing/1 -> Switch/2, Switch1/2, Out2/1  "reset"
  Sign2/1 -> Switch/3
  In3/1 -> Hit Crossing/1
  MinMax/1 -> Switch1/1
  Switch1/1 -> Product/2
  static friction [N]/1 -> Mux1/2
  Abs/1 -> MinMax/1

== system Modello_attuatore/Actuation System/Servovalve/Servovalve Dynamic/Torque Motor/Demagnetization ==
  In1 : Inport
  Add1 : Sum  Inputs=-|+
  Add2 : Sum  Inputs=+|+
  Add3 : Sum  Inputs=+|-
  Compare To Constant : simulink/Logic and Bit Operations/Compare To Constant  relop=>  const=0  OutDataTypeStr=uint8
  Constant1 : Constant
  Constant3 : Constant  Value=Temperature_threshold
  From File3 : FromFile  FileName=E10_temperature.mat  SampleTime=dt_sim
  Gain : Gain  Gain=2
  Gain1 : Gain  Gain=Resistance
  Integrator1 : Integrator  InitialCondition=demag0_1
  Math Function : Math  Operator=magnitude^2  SignedPower=on
  Product1 : Product  SaturateOnIntegerOverflow=on  OutDataTypeStr=Inherit: Same as first input
  Saturation : Saturate  UpperLimit=0.7  LowerLimit=0
  Thermal Resistence : Gain  Gain=R_th1
  To Workspace : ToWorkspace  VariableName=demag_size  SaveFormat=Structure With Time  SampleTime=-1
  amount of demagnetization : Gain  Gain=m_thermal
  transfer function : TransferFcn  Denominator=[tau_w1 1]
  Out2 : Outport
  wires:
  Gain/1 -> Math Function/1
  Math Function/1 -> Gain1/1
  Gain1/1 -> Thermal Resistence/1
  Thermal Resistence/1 -> Add2/2
  From File3/1 -> Add2/1
  Add2/1 -> transfer function/1
  In1/1 -> Gain/1
  Constant3/1 -> Add1/1
  transfer function/1 -> Add1/2
  Add1/1 -> Product1/1, Compare To Constant/1
  Compare To Constant/1 -> Product1/2
  Product1/1 -> Integrator1/1
  Integrator1/1 -> amount of demagnetization/1
  amount of demagnetization/1 -> Saturation/1
  Add3/1 -> Out2/1
  Constant1/1 -> Add3/1
  Saturation/1 -> Add3/2, To Workspace/1

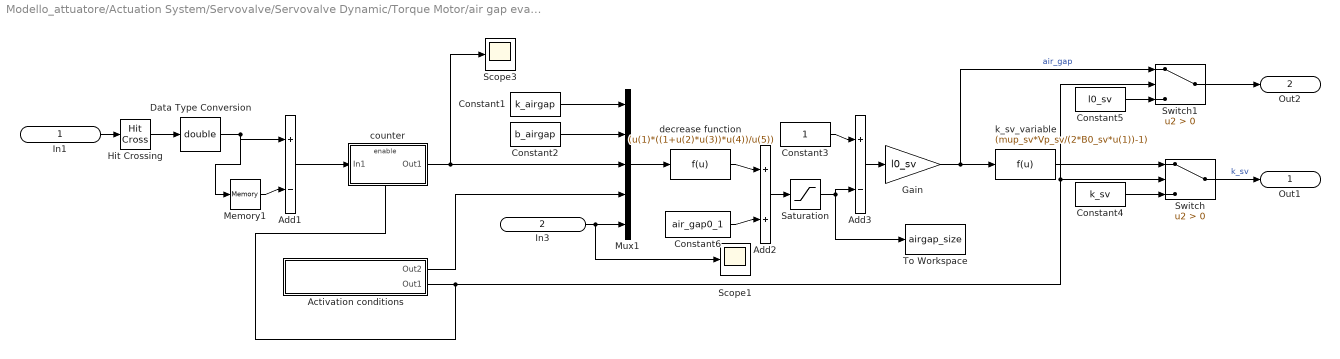
== system Modello_attuatore/Actuation System/Servovalve/Servovalve Dynamic/Torque Motor/air gap evaluation ==
  In1 : Inport
  In3 : Inport  Port=2
  Activation conditions : Subsystem
  Add1 : Sum  Inputs=+|-
  Add2 : Sum  Inputs=+|+
  Add3 : Sum  Inputs=+|-
  Constant1 : Constant  Value=k_airgap
  Constant2 : Constant  Value=b_airgap
  Constant3 : Constant
  Constant4 : Constant  Value=k_sv
  Constant5 : Constant  Value=l0_sv
  Constant6 : Constant  Value=air_gap0_1
  Data Type Conversion : DataTypeConversion  OutDataTypeStr=double  SaturateOnIntegerOverflow=off  RndMeth=Floor
  Gain : Gain  Gain=l0_sv
  Hit Crossing : HitCross
  Memory1 : Memory
  Mux1 : Mux  Inputs=5
  Saturation : Saturate  UpperLimit=0.65  LowerLimit=0
  Scope1 : Scope
  Scope3 : Scope
  Switch : Switch  Criteria=u2 > Threshold  SaturateOnIntegerOverflow=off  InputSameDT=off
  Switch1 : Switch  Criteria=u2 > Threshold  SaturateOnIntegerOverflow=off  InputSameDT=off
  To Workspace : ToWorkspace  VariableName=airgap_size  SaveFormat=Structure With Time  SampleTime=-1
  counter : Subsystem
  decrease function : Fcn  Expr=(u(1)*((1+u(2)*u(3))*u(4))/u(5))
  k_sv_variable : Fcn  Expr=(mup_sv*Vp_sv/(2*B0_sv*u(1))-1)
  Out1 : Outport
  Out2 : Outport  Port=2
  wires:
  Hit Crossing/1 -> Data Type Conversion/1
  Memory1/1 -> Add1/2
  Data Type Conversion/1 -> Add1/1, Memory1/1
  Add1/1 -> counter/1(In1)
  In1/1 -> Hit Crossing/1
  Mux1/1 -> decrease function/1
  Constant1/1 -> Mux1/1
  Constant2/1 -> Mux1/2
  Activation conditions/1(Out2) -> Mux1/4
  In3/1 -> Mux1/5, Scope1/1
  Add3/1 -> Gain/1
  Constant3/1 -> Add3/1
  Gain/1 -> k_sv_variable/1, Switch1/1  "air_gap"
  k_sv_variable/1 -> Switch/1
  Switch/1 -> Out1/1  "k_sv"
  Constant4/1 -> Switch/3
  Switch1/1 -> Out2/1
  Activation conditions/2(Out1) -> Switch/2, Switch1/2, counter/Enable
  Constant5/1 -> Switch1/3
  counter/1(Out1) -> Mux1/3, Scope3/1
  decrease function/1 -> Add2/1
  Constant6/1 -> Add2/2
  Saturation/1 -> Add3/2, To Workspace/1
  Add2/1 -> Saturation/1

== system Modello_attuatore/Actuation System/Servovalve/Spool/orifice1R-resistences/Cd ==
  In2 : Inport
  In1 : Inport  Port=2
  In3 : Inport  Port=3
  Abs : Abs  SaturateOnIntegerOverflow=off
  Fcn : Fcn  Expr=0.22*sqrt(log(1+u(1)))
  Fcn1 : Fcn  Expr=u(2)*(1+0.2*hr_sv/(u(1)+hr_sv))
  Fcn2 : Fcn  Expr=2*u(3)*u(2)/(u(4)*(wsp_sv+u(1)))
  Fcn3 : Fcn  Expr=(u(2)*(u(1)+u(3)))/(2*(u(1)*u(3)))
  Lookup Table1 : Lookup  InputValues=R_sp_C(1,:)  Table=R_sp_C(2,:)  SaturateOnIntegerOverflow=off
  Memory1 : Memory  InitialCondition=eps
  Mux1 : Mux  Inputs=2
  Mux2 : Mux  Inputs=3
  Mux3 : Mux  Inputs=3
  Product : Product  RndMeth=Zero
  Saturation : Saturate  UpperLimit=Remax_sv  LowerLimit=0
  Saturation1 : Saturate  UpperLimit=Cdmax_sv  LowerLimit=Cdmin_sv
  Scope2 : Scope  NumInputPorts=2
  gioco radiale2 : Constant  Value=rj_sv
  gioco radiale3 : Constant  Value=wsp_sv
  Out3 : Outport
  wires:
  Fcn2/1 -> Saturation/1
  Saturation/1 -> Fcn/1
  Fcn/1 -> Mux1/2  "Cd0"
  Mux1/1 -> Fcn1/1
  Fcn1/1 -> Saturation1/1  "Cd"
  In3/1 -> Mux2/1, Mux3/1  "l[m]"
  Memory1/1 -> Mux2/2
  In2/1 -> Memory1/1  "Q1R[m3/s]"
  Mux2/1 -> Fcn2/1
  In1/1 -> Abs/1  "x[m]"
  gioco radiale3/1 -> Mux3/3
  Lookup Table1/1 -> Product/2  "c'"
  Mux3/1 -> Fcn3/1
  gioco radiale2/1 -> Mux3/2
  Fcn3/1 -> Lookup Table1/1  "r/d0"
  Product/1 -> Scope2/2, Out3/1  "Cd"
  Saturation1/1 -> Product/1, Scope2/1  "Cd"
  Abs/1 -> Mux1/1
  [Fluid_properties_var] -> Mux2/3

== system Modello_attuatore/Actuation System/Servovalve/Spool/orifice1S-resistences/Cd ==
  In2 : Inport
  In1 : Inport  Port=2
  In3 : Inport  Port=3
  Abs : Abs  SaturateOnIntegerOverflow=off
  Fcn : Fcn  Expr=0.22*sqrt(log(1+u(1)))
  Fcn1 : Fcn  Expr=u(2)*(1+0.2*hr_sv/(u(1)+hr_sv))
  Fcn2 : Fcn  Expr=2*u(3)*u(2)/(u(4)*(wsp_sv+u(1)))
  Fcn3 : Fcn  Expr=(u(2)*(u(1)+u(3)))/(2*(u(1)*u(3)))
  Lookup Table1 : Lookup  InputValues=R_sp_C(1,:)  Table=R_sp_C(2,:)  SaturateOnIntegerOverflow=off
  Memory1 : Memory  InitialCondition=eps
  Mux1 : Mux  Inputs=2
  Mux2 : Mux  Inputs=3
  Mux3 : Mux  Inputs=3
  Product : Product  RndMeth=Zero
  Saturation : Saturate  UpperLimit=Remax_sv  LowerLimit=0
  Saturation1 : Saturate  UpperLimit=Cdmax_sv  LowerLimit=Cdmin_sv
  Scope2 : Scope  NumInputPorts=2
  gioco radiale2 : Constant  Value=rj_sv
  gioco radiale3 : Constant  Value=wsp_sv
  Out3 : Outport
  wires:
  Fcn2/1 -> Saturation/1
  Saturation/1 -> Fcn/1
  Fcn/1 -> Mux1/2  "Cd0"
  Mux1/1 -> Fcn1/1
  Fcn1/1 -> Saturation1/1  "Cd"
  In3/1 -> Mux2/1, Mux3/1  "l[m]"
  Memory1/1 -> Mux2/2
  In2/1 -> Memory1/1  "Q1R[m3/s]"
  Mux2/1 -> Fcn2/1
  In1/1 -> Abs/1  "x[m]"
  gioco radiale3/1 -> Mux3/3
  Lookup Table1/1 -> Product/2  "c'"
  Mux3/1 -> Fcn3/1
  gioco radiale2/1 -> Mux3/2
  Fcn3/1 -> Lookup Table1/1  "r/d0"
  Product/1 -> Scope2/2, Out3/1  "Cd"
  Saturation1/1 -> Product/1, Scope2/1  "Cd"
  Abs/1 -> Mux1/1
  [Fluid_properties_var] -> Mux2/3

== system Modello_attuatore/Actuation System/Servovalve/Spool/orifice2R-resistences/Cd ==
  In2 : Inport
  In1 : Inport  Port=2
  In3 : Inport  Port=3
  Abs : Abs  SaturateOnIntegerOverflow=off
  Fcn : Fcn  Expr=0.22*sqrt(log(1+u(1)))
  Fcn1 : Fcn  Expr=u(2)*(1+0.2*hr_sv/(u(1)+hr_sv))
  Fcn2 : Fcn  Expr=2*u(3)*u(2)/(u(4)*(wsp_sv+u(1)))
  Fcn3 : Fcn  Expr=(u(2)*(u(1)+u(3)))/(2*(u(1)*u(3)))
  Lookup Table1 : Lookup  InputValues=R_sp_C(1,:)  Table=R_sp_C(2,:)  SaturateOnIntegerOverflow=off
  Memory1 : Memory  InitialCondition=eps
  Mux1 : Mux  Inputs=2
  Mux2 : Mux  Inputs=3
  Mux3 : Mux  Inputs=3
  Product : Product  RndMeth=Zero
  Saturation : Saturate  UpperLimit=Remax_sv  LowerLimit=0
  Saturation1 : Saturate  UpperLimit=Cdmax_sv  LowerLimit=Cdmin_sv
  Scope2 : Scope  NumInputPorts=2
  gioco radiale2 : Constant  Value=rj_sv
  gioco radiale3 : Constant  Value=wsp_sv
  Out3 : Outport
  wires:
  Fcn2/1 -> Saturation/1
  Saturation/1 -> Fcn/1
  Fcn/1 -> Mux1/2  "Cd0"
  Mux1/1 -> Fcn1/1
  Fcn1/1 -> Saturation1/1  "Cd"
  In3/1 -> Mux2/1, Mux3/1  "l[m]"
  Memory1/1 -> Mux2/2
  In2/1 -> Memory1/1  "Q1R[m3/s]"
  Mux2/1 -> Fcn2/1
  In1/1 -> Abs/1  "x[m]"
  gioco radiale3/1 -> Mux3/3
  Lookup Table1/1 -> Product/2  "c'"
  Mux3/1 -> Fcn3/1
  gioco radiale2/1 -> Mux3/2
  Fcn3/1 -> Lookup Table1/1  "r/d0"
  Product/1 -> Scope2/2, Out3/1  "Cd"
  Saturation1/1 -> Product/1, Scope2/1  "Cd"
  Abs/1 -> Mux1/1
  [Fluid_properties_var] -> Mux2/3

== system Modello_attuatore/Actuation System/Servovalve/Spool/orifice2S-resistences/Cd ==
  In2 : Inport
  In1 : Inport  Port=2
  In3 : Inport  Port=3
  Abs : Abs  SaturateOnIntegerOverflow=off
  Fcn : Fcn  Expr=0.22*sqrt(log(1+u(1)))
  Fcn1 : Fcn  Expr=u(2)*(1+0.2*hr_sv/(u(1)+hr_sv))
  Fcn2 : Fcn  Expr=2*u(3)*u(2)/(u(4)*(wsp_sv+u(1)))
  Fcn3 : Fcn  Expr=(u(2)*(u(1)+u(3)))/(2*(u(1)*u(3)))
  Lookup Table1 : Lookup  InputValues=R_sp_C(1,:)  Table=R_sp_C(2,:)  SaturateOnIntegerOverflow=off
  Memory1 : Memory  InitialCondition=eps
  Mux1 : Mux  Inputs=2
  Mux2 : Mux  Inputs=3
  Mux3 : Mux  Inputs=3
  Product : Product  RndMeth=Zero
  Saturation : Saturate  UpperLimit=Remax_sv  LowerLimit=0
  Saturation1 : Saturate  UpperLimit=Cdmax_sv  LowerLimit=Cdmin_sv
  Scope2 : Scope  NumInputPorts=2
  gioco radiale2 : Constant  Value=rj_sv
  gioco radiale3 : Constant  Value=wsp_sv
  Out3 : Outport
  wires:
  Fcn2/1 -> Saturation/1
  Saturation/1 -> Fcn/1
  Fcn/1 -> Mux1/2  "Cd0"
  Mux1/1 -> Fcn1/1
  Fcn1/1 -> Saturation1/1  "Cd"
  In3/1 -> Mux2/1, Mux3/1  "l[m]"
  Memory1/1 -> Mux2/2
  In2/1 -> Memory1/1  "Q1R[m3/s]"
  Mux2/1 -> Fcn2/1
  In1/1 -> Abs/1  "x[m]"
  gioco radiale3/1 -> Mux3/3
  Lookup Table1/1 -> Product/2  "c'"
  Mux3/1 -> Fcn3/1
  gioco radiale2/1 -> Mux3/2
  Fcn3/1 -> Lookup Table1/1  "r/d0"
  Product/1 -> Scope2/2, Out3/1  "Cd"
  Saturation1/1 -> Product/1, Scope2/1  "Cd"
  Abs/1 -> Mux1/1
  [Fluid_properties_var] -> Mux2/3

== system Modello_attuatore/Actuation System/Servovalve/Servovalve Dynamic/Jet pipe dynamic/Double Integrator/Limit ==
  In2 : Inport
  In1 : Inport  Port=2
  Constant : Constant
  Constant1 : Constant  Value=-1
  Constant2 : Constant  Value=0
  Constant3 : Constant  Value=0
  Logical Operator : Logic  AllPortsSameDT=off
  Logical Operator1 : Logic  AllPortsSameDT=off
  Logical Operator2 : Logic  Operator=NOR  AllPortsSameDT=off
  Product : Product  RndMeth=Zero
  Relational Operator : RelationalOperator  Operator=>  OutDataTypeStr=boolean  InputSameDT=off
  Relational Operator1 : RelationalOperator  Operator===  OutDataTypeStr=boolean  InputSameDT=off
  Relational Operator2 : RelationalOperator  Operator=<  OutDataTypeStr=boolean  InputSameDT=off
  Relational Operator3 : RelationalOperator  Operator===  OutDataTypeStr=boolean  InputSameDT=off
  Out2 : Outport
  wires:
  In2/1 -> Relational Operator/1, Product/1, Relational Operator2/1  "xrod_dd [m/s2]"
  In1/1 -> Relational Operator3/1, Relational Operator1/1  "limit xrod"
  Constant3/1 -> Relational Operator/2
  Constant/1 -> Relational Operator1/2
  Constant1/1 -> Relational Operator3/2
  Constant2/1 -> Relational Operator2/2
  Relational Operator/1 -> Logical Operator/1
  Relational Operator1/1 -> Logical Operator/2
  Relational Operator3/1 -> Logical Operator1/1
  Relational Operator2/1 -> Logical Operator1/2
  Logical Operator/1 -> Logical Operator2/1
  Logical Operator1/1 -> Logical Operator2/2
  Logical Operator2/1 -> Product/2
  Product/1 -> Out2/1  "xrod_dd [m2/s]"

== system Modello_attuatore/Actuation System/Servovalve/Servovalve Dynamic/Spool  dynamic/Double Integrator/Limit ==
  In2 : Inport
  In1 : Inport  Port=2
  Constant : Constant
  Constant1 : Constant  Value=-1
  Constant2 : Constant  Value=0
  Constant3 : Constant  Value=0
  Logical Operator : Logic  AllPortsSameDT=off
  Logical Operator1 : Logic  AllPortsSameDT=off
  Logical Operator2 : Logic  Operator=NOR  AllPortsSameDT=off
  Product : Product  RndMeth=Zero
  Relational Operator : RelationalOperator  Operator=>  OutDataTypeStr=boolean  InputSameDT=off
  Relational Operator1 : RelationalOperator  Operator===  OutDataTypeStr=boolean  InputSameDT=off
  Relational Operator2 : RelationalOperator  Operator=<  OutDataTypeStr=boolean  InputSameDT=off
  Relational Operator3 : RelationalOperator  Operator===  OutDataTypeStr=boolean  InputSameDT=off
  Out2 : Outport
  wires:
  In2/1 -> Relational Operator/1, Product/1, Relational Operator2/1  "xrod_dd [m/s2]"
  In1/1 -> Relational Operator3/1, Relational Operator1/1  "limit xrod"
  Constant3/1 -> Relational Operator/2
  Constant/1 -> Relational Operator1/2
  Constant1/1 -> Relational Operator3/2
  Constant2/1 -> Relational Operator2/2
  Relational Operator/1 -> Logical Operator/1
  Relational Operator1/1 -> Logical Operator/2
  Relational Operator3/1 -> Logical Operator1/1
  Relational Operator2/1 -> Logical Operator1/2
  Logical Operator/1 -> Logical Operator2/1
  Logical Operator1/1 -> Logical Operator2/2
  Logical Operator2/1 -> Product/2
  Product/1 -> Out2/1  "xrod_dd [m2/s]"

== system Modello_attuatore/Actuation System/Servovalve/Servovalve Dynamic/Spool  dynamic/Flow Force/Q_max evaluation and flow angle variation ==
  In1 : Inport
  In2 : Inport  Port=2
  In3 : Inport  Port=3
  Constant3 : Constant  Value=Cdmin_sv
  Product3 : Product
  Product4 : Product
  Total Passage Area : Subsystem
  Variation of flow angle Q1 : Subsystem
  Variation of flow angle Q2 : Subsystem
  sqrt(0.5*dP/ro) : Fcn  Expr=sqrt(0.5*(u(1)-u(2))/u(3))
  cos(teta) of Q1 : Outport
  cos(teta) of Q2 : Outport  Port=2
  wires:
  Constant3/1 -> Product3/2
  sqrt(0.5*dP/ro)/1 -> Product4/1
  Total Passage Area/1(Out3) -> Product3/1
  Product3/1 -> Product4/2
  Product4/1 -> Variation of flow angle Q1/2(In3), Variation of flow angle Q2/1(In3)  "Q_max [m3/s]"
  Variation of flow angle Q1/1(cos(teta)) -> cos(teta) of Q1/1
  In1/1 -> Variation of flow angle Q1/1(In1)
  Variation of flow angle Q2/1(cos(teta)) -> cos(teta) of Q2/1
  In2/1 -> sqrt(0.5*dP/ro)/1
  In3/1 -> Variation of flow angle Q2/2(In1)

== system Modello_attuatore/Actuation System/Servovalve/Servovalve Dynamic/Torque Motor/air gap evaluation/Activation conditions ==
  Add1 : Sum  Inputs=+|-
  Add2 : Sum  Inputs=+|+
  Clock : Clock
  Compare To Constant : simulink/Logic and Bit Operations/Compare To Constant  relop=>  const=0  OutDataTypeStr=uint8
  Constant1 : Constant  Value=air_gap_fault_time
  Constant2 : Constant  Value=first_cycle-1
  Constant3 : Constant  Value=flight_hours
  Gain1 : Gain  Gain=flight_hours/364
  Product1 : Product  SaturateOnIntegerOverflow=on  OutDataTypeStr=Inherit: Same as first input
  Product2 : Product  SaturateOnIntegerOverflow=on  OutDataTypeStr=Inherit: Same as first input
  Relational Operator : RelationalOperator  Operator=<  OutDataTypeStr=boolean  InputSameDT=off
  Saturation : Saturate  UpperLimit=inf  LowerLimit=0
  Out2 : Outport
  Out1 : Outport  Port=2
  tag scope: flight_time=global
  wires:
  Constant2/1 -> Saturation/1
  Constant3/1 -> Product2/2
  Product2/1 -> Add2/1
  Clock/1 -> Gain1/1
  Gain1/1 -> Add2/2
  Constant1/1 -> Relational Operator/1, Add1/2
  Add2/1 -> Relational Operator/2, Add1/1, [flight_time]  "flight time [h]"
  Relational Operator/1 -> Out1/1  "enable_com"
  Add1/1 -> Compare To Constant/1, Product1/1
  Compare To Constant/1 -> Product1/2
  Product1/1 -> Out2/1  "flight time [h]"
  Saturation/1 -> Product2/1

== system Modello_attuatore/Actuation System/Servovalve/Servovalve Dynamic/Torque Motor/air gap evaluation/counter ==
  In1 : Inport
  Enable : EnablePort
  Add2 : Sum  Inputs=+|+
  Compare To Constant : simulink/Logic and Bit Operations/Compare To Constant  relop=>  const=0  OutDataTypeStr=uint8
  Data Type Conversion1 : DataTypeConversion  OutDataTypeStr=double  SaturateOnIntegerOverflow=off  RndMeth=Floor
  Memory : Memory
  Out1 : Outport
  wires:
  Add2/1 -> Memory/1, Out1/1
  Compare To Constant/1 -> Data Type Conversion1/1
  In1/1 -> Compare To Constant/1
  Memory/1 -> Add2/2
  Data Type Conversion1/1 -> Add2/1

== system Modello_attuatore/Actuation System/Servovalve/Servovalve Dynamic/Spool  dynamic/Flow Force/Q_max evaluation and flow angle variation/Total Passage Area ==
  note: Xvr1 +Xvr2
  note: Xvs1 +Xvs2
  Add1 : Sum  Inputs=-|+
  Add2 : Sum  Inputs=+|-
  Add3 : Sum  Inputs=-|+
  Add4 : Sum  Inputs=+|-
  Add5 : Sum  Inputs=+|+
  Add6 : Sum  Inputs=+|+
  Add7 : Sum  Inputs=+|+
  Constant3 : Constant  Value=xspmax_sv
  Gain : Gain  Gain=0.5
  MinMax{,1..3} (4 alike) : MinMax  Inputs=2
  Product : Product
  Product1 : Product
  gioco radiale1 : Constant  Value=wsp_sv
  ricoprimento : Constant  Value=OV_S1
  ricoprimento1 : Constant  Value=OV_S2
  ricoprimento2 : Constant  Value=OV_R1
  ricoprimento3 : Constant  Value=OV_R2
  Out3 : Outport
  wires:
  ricoprimento/1 -> Add3/1
  Constant3/1 -> Add2/1, Add1/2, Add3/2, MinMax1/2, MinMax/1, Add4/1, MinMax3/1, MinMax2/2
  ricoprimento1/1 -> Add1/1
  ricoprimento2/1 -> Add2/2
  ricoprimento3/1 -> Add4/2
  Add6/1 -> Product/1
  gioco radiale1/1 -> Product1/1, Product/2
  Add5/1 -> Product1/2
  Product1/1 -> Add7/2  "A_VR"
  Product/1 -> Add7/1  "A_VS"
  Add7/1 -> Gain/1
  Gain/1 -> Out3/1  "A_median"
  Add1/1 -> MinMax/2
  Add3/1 -> MinMax1/1
  MinMax/1 -> Add6/2
  MinMax1/1 -> Add6/1
  Add4/1 -> MinMax3/2
  Add2/1 -> MinMax2/1
  MinMax2/1 -> Add5/1
  MinMax3/1 -> Add5/2

== system Modello_attuatore/Actuation System/Servovalve/Servovalve Dynamic/Spool  dynamic/Flow Force/Q_max evaluation and flow angle variation/Variation of flow angle Q1 ==
  In1 : Inport
  In3 : Inport  Port=2
  Constant4 : Constant  Value=0.5
  Flow less than 0.05 : Fcn  Expr=1-10*u(1)
  Product5 : Product  Inputs=*/  SaturateOnIntegerOverflow=on  OutDataTypeStr=Inherit: Same as first input
  Switch : Switch  Criteria=u2 > Threshold  Threshold=0.05  SaturateOnIntegerOverflow=off  InputSameDT=off
  cos(teta) : Outport
  wires:
  Switch/1 -> cos(teta)/1
  Constant4/1 -> Switch/1
  Product5/1 -> Flow less than 0.05/1, Switch/2
  In1/1 -> Product5/1
  In3/1 -> Product5/2
  Flow less than 0.05/1 -> Switch/3
